simulink model "model_1D"  (R2016a)
settings: Solver=FixedStepAuto  StartTime=0.0  StopTime=10.0  FixedStep=0.001  RelTol=1e-3
InitFcn:
  | initCallback_model1D
values from neighbouring files (symbols this model uses):
  C_phi = 1    [initCallback_model1D.m]
  C_psi = 2    [initCallback_model1D.m]
  g = 9.81    [initCallback_model1D.m]
  l_AB = 3    [initCallback_model1D.m]
  l_AC = 4    [initCallback_model1D.m]
  m_K = 5    [initCallback_model1D.m]
  m_R = 1    [initCallback_model1D.m]
  O_A_K = 2    [initCallback_model1D.m]
  O_B_R = 3    [initCallback_model1D.m]
  phi_0 = degtorad(3)    [initCallback_model1D.m]
  phi__d_0 = 0    [initCallback_model1D.m]
  psi_0 = 0    [initCallback_model1D.m]
  psi__d_0 = 0    [initCallback_model1D.m]
  T_M = 5    [initCallback_model1D.m]
  T_M_e = 5.5e-4    (= 0.00055)    [initCallback_model1D.m]
  T_M_m = 12.4e-3    (= 0.0124)    [initCallback_model1D.m]
settings Model: Creator=ich  LastModifiedBy=ich

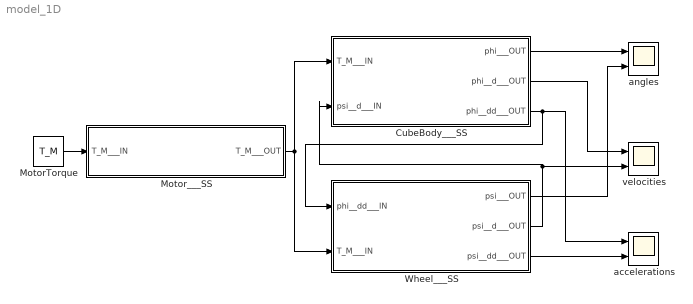
== system model_1D ==
  CubeBody___SS : Subsystem
  MotorTorque : Constant  Value=T_M
  Motor___SS : Subsystem
  Wheel___SS : Subsystem
  accelerations : Scope  NumInputPorts=2
  angles : Scope  NumInputPorts=2
  velocities : Scope  NumInputPorts=2
  wires:
  Motor___SS/1(T_M___OUT) -> Wheel___SS/2(T_M___IN), CubeBody___SS/1(T_M___IN)
  Wheel___SS/2(psi__d___OUT) -> CubeBody___SS/2(psi__d___IN), velocities/2
  CubeBody___SS/3(phi__dd___OUT) -> accelerations/1, Wheel___SS/1(phi__dd___IN)
  CubeBody___SS/1(phi___OUT) -> angles/1
  Wheel___SS/1(psi___OUT) -> angles/2
  CubeBody___SS/2(phi__d___OUT) -> velocities/1
  Wheel___SS/3(psi__dd___OUT) -> accelerations/2
  MotorTorque/1 -> Motor___SS/1(T_M___IN)

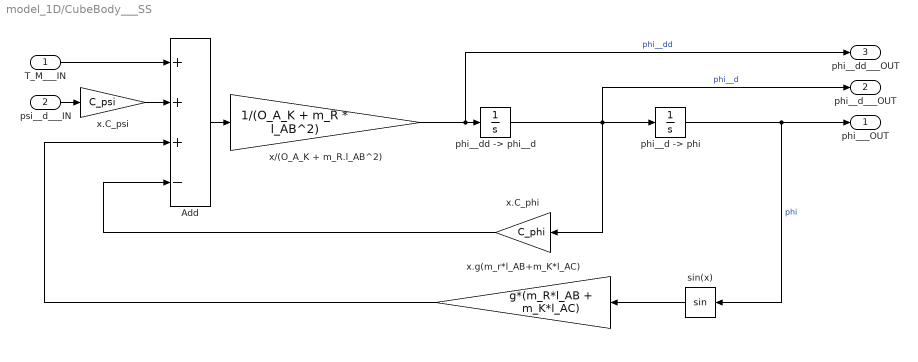
== system model_1D/CubeBody___SS ==
  T_M___IN : Inport
  psi__d___IN : Inport  Port=2
  Add : Sum  Inputs=+++-
  "phi__d -> phi" : Integrator  InitialCondition=phi_0
  "phi__dd -> phi__d" : Integrator  InitialCondition=phi__d_0
  sin(x) : Trigonometry
  x.C_phi : Gain  Gain=C_phi
  x.C_psi : Gain  Gain=C_psi
  x.g(m_r*l_AB+m_K*l_AC) : Gain  Gain=g*(m_R*l_AB + m_K*l_AC)
  x/(O_A_K + m_R.l_AB^2) : Gain  Gain=1/(O_A_K + m_R * l_AB^2)
  phi___OUT : Outport
  phi__d___OUT : Outport  Port=2
  phi__dd___OUT : Outport  Port=3
  wires:
  "phi__d -> phi"/1 -> sin(x)/1, phi___OUT/1  "phi"
  "phi__dd -> phi__d"/1 -> x.C_phi/1, phi__d___OUT/1, "phi__d -> phi"/1  "phi__d"
  x/(O_A_K + m_R.l_AB^2)/1 -> phi__dd___OUT/1, "phi__dd -> phi__d"/1  "phi__dd"
  Add/1 -> x/(O_A_K + m_R.l_AB^2)/1
  T_M___IN/1 -> Add/1
  psi__d___IN/1 -> x.C_psi/1
  x.C_psi/1 -> Add/2
  sin(x)/1 -> x.g(m_r*l_AB+m_K*l_AC)/1
  x.g(m_r*l_AB+m_K*l_AC)/1 -> Add/3
  x.C_phi/1 -> Add/4

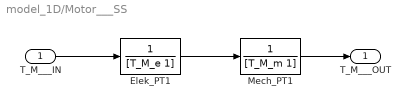
== system model_1D/Motor___SS ==
  T_M___IN : Inport
  Elek_PT1 : TransferFcn  Denominator=[T_M_e 1]
  Mech_PT1 : TransferFcn  Denominator=[T_M_m 1]
  T_M___OUT : Outport
  wires:
  T_M___IN/1 -> Elek_PT1/1
  Elek_PT1/1 -> Mech_PT1/1
  Mech_PT1/1 -> T_M___OUT/1

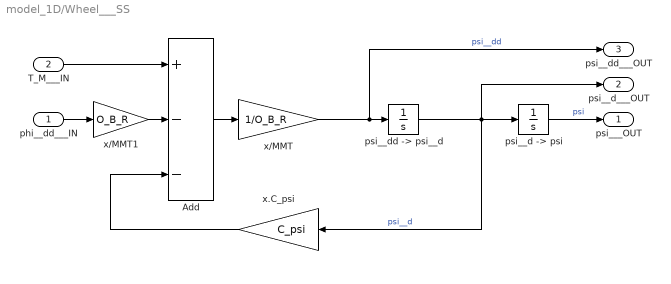
== system model_1D/Wheel___SS ==
  phi__dd___IN : Inport
  T_M___IN : Inport  Port=2
  Add : Sum  Inputs=+--
  "psi__d -> psi" : Integrator  InitialCondition=psi_0
  "psi__dd -> psi__d" : Integrator  InitialCondition=psi__d_0
  x.C_psi : Gain  Gain=C_psi
  x/MMT : Gain  Gain=1/O_B_R
  x/MMT1 : Gain  Gain=O_B_R
  psi___OUT : Outport
  psi__d___OUT : Outport  Port=2
  psi__dd___OUT : Outport  Port=3
  wires:
  "psi__d -> psi"/1 -> psi___OUT/1  "psi"
  "psi__dd -> psi__d"/1 -> psi__d___OUT/1, "psi__d -> psi"/1, x.C_psi/1  "psi__d"
  x/MMT/1 -> psi__dd___OUT/1, "psi__dd -> psi__d"/1  "psi__dd"
  Add/1 -> x/MMT/1
  T_M___IN/1 -> Add/1
  x.C_psi/1 -> Add/3
  phi__dd___IN/1 -> x/MMT1/1
  x/MMT1/1 -> Add/2
